simulink model "HQEV_MiL_20160830_integrate"  (Simulink 8.3)
settings: Solver=FixedStepDiscrete  StartTime=0.0  StopTime=inf  FixedStep=0.01  RelTol=1e-3
PostLoadFcn:
  | , if any(exist('dsrtsu_mdlpostloadfcn', 'file') == [2, 3, 6]), try dsrtsu_mdlpostloadfcn('Execute', bdroot); catch fprintf('Error in PostLoadFcn (dsrtsu_mdlpostloadfcn) for model "%s":\n %s\n', bdroot, lasterr); end, end,
values from neighbouring files (symbols this model uses):
  Bat_C_Ah = 36    [parameter_V1.mat]
  Bat_ocv_xIndex = [5 10 20 30 40 50 60 70 80 90 95]    [parameter_V1.mat]
  Bat_ocv_z = [329 332 340 345 347 351 358 372 377 386 391]    [parameter_V1.mat]
  Bat_R_ohm_z = [4.41 3.46 1.57 1.07 0.76 0.63 0.55 0.44 0.41 0.4 0.4 3.14 ... (66 elements, 11x6)]    [parameter_V1.mat]
  Bat_SOC_Init = 90    [parameter_V1.mat]
  Env_hum_pct_Ambient = 30    [parameter_V1.mat]
  Env_Slope_deg = 0    [parameter_V1.mat]
  Env_Temp_degC_Ambient = 25    [parameter_V1.mat]
  Env_v_kmph_HWind = 0    [parameter_V1.mat]
  Reducer_F_i = 7.23    [parameter_V1.mat]
  Reducer_R_i = 7.23    [parameter_V1.mat]
  Veh =     [parameter_V1.mat]
  Veh_A_m2_Fr = 2.246    [parameter_V1.mat]
  Veh_F_Brake =     [parameter_V1.mat]
  Veh_fac_AirDrag = 0.326    [parameter_V1.mat]
  Veh_fac_WhDragFrict_0 = 0.011    [parameter_V1.mat]
  Veh_g_mps2_C = 9.81    [parameter_V1.mat]
  Veh_GainBrake =     [parameter_V1.mat]
  Veh_h_m_COGHigh = 0.5    [parameter_V1.mat]
  Veh_J_kgm2_Wh = 1.3635    [parameter_V1.mat]
  Veh_L_m_AxlBas = 2.63    [parameter_V1.mat]
  Veh_M_kg = 1427    [parameter_V1.mat]
  Veh_mu_Brake = 0.4    [parameter_V1.mat]
  Veh_mu_Tyre =     [parameter_V1.mat]
  Veh_num_FrictPair = 8    [parameter_V1.mat]
  Veh_pct_Brk = 70    [parameter_V1.mat]
  Veh_r_dyn =     [parameter_V1.mat]
  Veh_r_m_BrkDisk = 0.136    [parameter_V1.mat]
  Veh_rho_kgpm3_Air = 1.2258    [parameter_V1.mat]
undefined symbols (not defined in the file or in its folder): DiscIntNeverNeededParam, p_bool_False_M, p_bool_True_M
libraries: BaseOperationLib_Browser x38, simulink x9, DTQC_lib x1, ERR_lib x1, MQM_lib x1, PTCL_lib x1, PUD_lib x1, TQD_lib x1, TQR_lib x1, VMM_lib x1, ACCA_lib x1, BBCA_lib x1
(part 6 of 15)

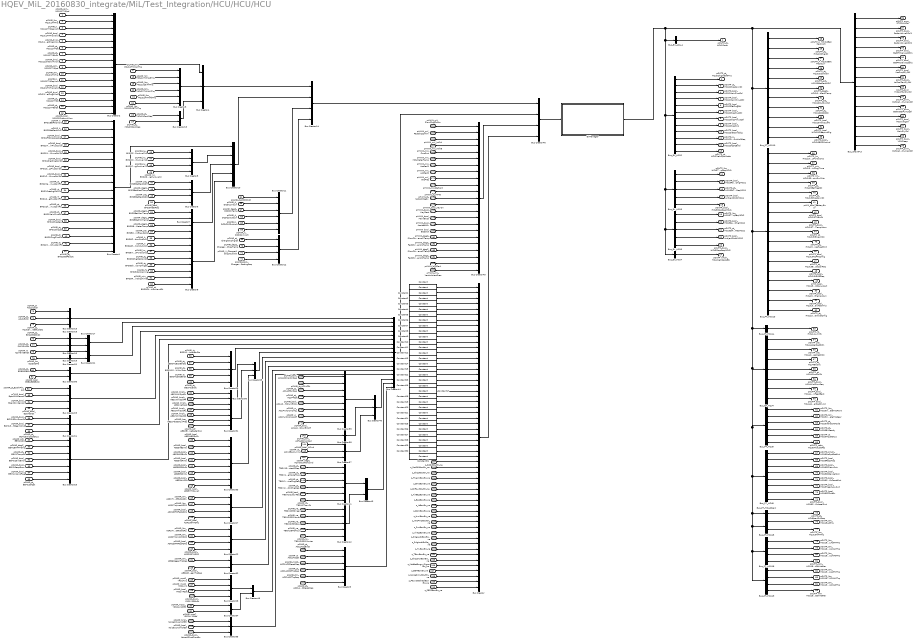
== system HQEV_MiL_20160830_integrate/MiL/Test_Integration/HCU/HCU/HCU ==
  pCANR_rpm_MCU11TMSpd : Inport
  pCANR_Nm_MCU11TMTrq : Inport  Port=2
  pCANR_V_MCU11TMCapVolt : Inport  Port=3
  pCANR_bool_MCU11TMTrqValid : Inport  Port=4
  pCANR_bool_MCU11PreChrgAllow : Inport  Port=5
  pCANR_st_MCU11TMSt : Inport  Port=6
  pCANR_st_MCU11TMErrSt : Inport  Port=7
  pCANR_bool_MCU11ShtdwnAllow : Inport  Port=8
  pCANR_rpm_MCU21TMSpd : Inport  Port=9
  pCANR_Nm_MCU21TMTrq : Inport  Port=10
  pCANR_V_MCU21TMCapVolt : Inport  Port=11
  pCANR_bool_MCU21TMTrqValid : Inport  Port=12
  pCANR_bool_MCU21PreChrgAllow : Inport  Port=13
  pCANR_st_MCU21TMSt : Inport  Port=14
  pCANR_st_MCU21TMErrSt : Inport  Port=15
  pCANR_bool_MCU21ShtdwnAllow : Inport  Port=16
  pCANR_Nm_MCU12TMMAMTrq : Inport  Port=17
  pCANR_Nm_MCU12TMMAGTrq : Inport  Port=18
  pCANR_Nm_MCU12CalTMTrq : Inport  Port=19
  pCANR_Nm_MCU22TMMAMTrq : Inport  Port=20
  pCANR_Nm_MCU22TMMAGTrq : Inport  Port=21
  pCANR_Nm_MCU22CalTMTrq : Inport  Port=22
  pCANR_st_MCU13CoolReq : Inport  Port=23
  pCANR_st_MCU23CoolReq : Inport  Port=24
  pCANR_V_BMS1BatPackVolt : Inport  Port=25
  pCANR_A_BMS1BatPackCurr : Inport  Port=26
  pCANR_bool_BMS1FltDisposeSig : Inport  Port=27
  pCANR_bool_BMS1MainPlusCoilSt : Inport  Port=28
  pCANR_bool_BMS1MainMinusCoilSt : Inport  Port=29
  pCANR_bool_BMS1PreChrgCoilSt : Inport  Port=30
  pCANR_bool_BMS1ChrgPlusCoilSt : Inport  Port=31
  pCANR_bool_BMS1ChrgMinusCoilSt : Inport  Port=32
  pCANR_st_BMS1MainMinusCoilFlt : Inport  Port=33
  pCANR_st_BMS1PrechrgCoilFlt : Inport  Port=34
  pCANR_st_BMS1ChrgPlusCoilFlt : Inport  Port=35
  pCANR_st_BMS1ChrgMinusCoilFlt : Inport  Port=36
  pCANR_st_BMS1MainPlusFlt : Inport  Port=37
  pCANR_bool_BMS1ChrgReq : Inport  Port=38
  pCANR_st_BMS1ChrgSt : Inport  Port=39
  pCANR_st_BMS1ChrgPlusFlt : Inport  Port=40
  pCANR_st_BMS1MainPlusCoilFlt : Inport  Port=41
  pCANR_st_BMS1BatPackSt : Inport  Port=42
  pCANR_kw_BMS2ChrgPwrAvail10 : Inport  Port=43
  pCANR_kw_BMS2DischrgPwrAvail10 : Inport  Port=44
  pCANR_kw_BMS2ChrgPwrAvail2 : Inport  Port=45
  pCANR_kw_BMS2DischrgPwrAvail2 : Inport  Port=46
  pCANR_pct_BMS3BatPackSOH : Inport  Port=47
  pCANR_degC_BMS3BatPackTemp : Inport  Port=48
  pCANR_pct_BMS3BatPackSOC : Inport  Port=49
  pCANR_bool_BMS3HeatReq : Inport  Port=50
  pCANR_degC_BMS5BatMaxTemp : Inport  Port=51
  pCANR_degC_BMS5BatMinTemp : Inport  Port=52
  pCANR_degC_BMS5BatInWaterTemp : Inport  Port=53
  pCANR_pct_BMS5RemainEngyRatio : Inport  Port=54
  pCANR_A_BMS6ChrgStationOutCurr : Inport  Port=55
  pCANR_V_BMS6ChrgStationOutVolt : Inport  Port=56
  pCANR_kw_BMS6InstnsPwrCnsmp : Inport  Port=57
  pCANR_st_BMS5ChrgStationSt : Inport  Port=58
  pCANR_st_BMS6ChrgStationCnfigSt : Inport  Port=59
  pCANR_st_BMS5IslaWarning : Inport  Port=60
  pCANR_min_BMS5RemainChrgTime : Inport  Port=61
  pCANR_st_BMS5ChrgStationHandSt : Inport  Port=62
  pCANR_A_DCDC1OutCurr : Inport  Port=63
  pCANR_st_DCDC1St : Inport  Port=64
  pCANR_V_DCDC1COutVolt : Inport  Port=65
  pCANR_A_DCDC1InCurr : Inport  Port=66
  pCANR_degC_DCDC1Temp : Inport  Port=67
  pCANR_V_DCDC1InVolt : Inport  Port=68
  pCANR_st_Charger1ChrgrSt : Inport  Port=69
  pCANR_degC_Charger1ChrgrTemp : Inport  Port=70
  pCANR_V_Charger1ChrgrOutVolt : Inport  Port=71
  pCANR_bool_Charger1RechrgReq : Inport  Port=72
  pCANR_st_ACU1Crash : Inport  Port=73
  pCANR_st_ACU1ErrSt : Inport  Port=74
  pCANR_st_ACU1DrvSideBuckSts : Inport  Port=75
  pCANR_st_EPS1EPSErrSt : Inport  Port=76
  pCANR_st_SAS1SASSt : Inport  Port=77
  pCANR_st_IC1HandBrkSt : Inport  Port=78
  pCANR_km_IC2DDSPS : Inport  Port=79
  pCANR_st_EPB1EPBSt : Inport  Port=80
  pCANR_bool_EPB1EPBErrSt : Inport  Port=81
  pCANR_st_EparkPrkLock : Inport  Port=82
  pCANR_bool_EparkPrkSensor : Inport  Port=83
  pCANR_bool_EparkDrvSensor : Inport  Port=84
  pCANR_bool_EparkErrSt : Inport  Port=85
  pCANR_bool_BCM13DrvDoorSt : Inport  Port=86
  pCANR_bool_BCM13HighBeamCmd : Inport  Port=87
  pCANR_st_BCM13WiperStatus : Inport  Port=88
  pCANR_pct_EEM1SOC : Inport  Port=89
  pCANR_degC_EEM1BATTTemp : Inport  Port=90
  pCANR_st_EEM1TempSt : Inport  Port=91
  pCANR_bool_EEM1CalibError : Inport  Port=92
  pCANR_bool_EEM1RespError : Inport  Port=93
  pCANR_bool_EEM1InconsFlag : Inport  Port=94
  pCANR_st_EEM1SOCSt : Inport  Port=95
  pCANR_st_EGSM1PrkLockBtnSts : Inport  Port=96
  pCANR_st_EGSM1EcoBtnSts : Inport  Port=97
  pCANR_st_EGSM1SBW1LvlPstn : Inport  Port=98
  pCANR_st_EGSM1SecBtnSt : Inport  Port=99
  pCANR_st_EGSM1ErrSt : Inport  Port=100
  pCANR_kmph_ABS1WhlSpdFL : Inport  Port=101
  pCANR_kmph_ABS1WhlSpdFR : Inport  Port=102
  pCANR_kmph_ABS1VehSpd : Inport  Port=103
  pCANR_kmph_ABS2WhlSpdRL : Inport  Port=104
  pCANR_kmph_ABS2WhlSpdRR : Inport  Port=105
  pCANR_bar_ABS2MasterCylPres : Inport  Port=106
  pCANR_pct_ABS2BrakePedalPos : Inport  Port=107
  pCANR_bool_ABS3ABSErrSt : Inport  Port=108
  pCANR_bool_ABS3ABSIntv : Inport  Port=109
  pCANR_bool_ABS3ASRErrSt : Inport  Port=110
  pCANR_bool_ABS3ASRIntv : Inport  Port=111
  pCANR_bool_ABS3ESPErrSt : Inport  Port=112
  pCANR_bool_ABS3ESPIntv : Inport  Port=113
  pCANR_bool_ABS3HHCSt : Inport  Port=114
  pCANR_bool_ABS3HHCAvail : Inport  Port=115
  pCANR_Nm_ASR1TrqRdctFastASR1 : Inport  Port=116
  pCANR_Nm_ASR1TrqIncrsMSR1 : Inport  Port=117
  pCANR_bool_ASR1StTRFastASR1 : Inport  Port=118
  pCANR_bool_ASR1StTIMSR1 : Inport  Port=119
  pCANR_Nm_ASR2TrqRdctFastASR2 : Inport  Port=120
  pCANR_Nm_ASR2TrqIncrsMSR2 : Inport  Port=121
  pCANR_bool_ASR2StTRFastASR2 : Inport  Port=122
  pCANR_bool_ASR2StTIMSR2 : Inport  Port=123
  pCANR_Nm_ABS6RegenTrqReq : Inport  Port=124
  pCANR_bool_ABS6StRegenTrqReq : Inport  Port=125
  pCANR_mps2_YRS1AX1 : Inport  Port=126
  pCANR_mps2_YRS1AY1 : Inport  Port=127
  pCANR_bool_YRS1YRSSt : Inport  Port=128
  pCANR_bool_YRS1YRSErrSt : Inport  Port=129
  pCANR_mps2_YRS2AX1Ofst : Inport  Port=130
  pCANR_mps2_YRS2AY1Ofst : Inport  Port=131
  pCANR_bool_Noise1OverVoltErr : Inport  Port=132
  pCANR_bool_Noise1UndrVoltErr : Inport  Port=133
  pCANR_bool_Noise1ShotCicutErr : Inport  Port=134
  pCANR_bool_AC1ACCmprOnReq : Inport  Port=135
  pCANR_st_AC1ACSt : Inport  Port=136
  pCANR_st_AC1ACFanReq : Inport  Port=137
  pCANR_st_AC1PTCSt : Inport  Port=138
  pCANR_bool_AC1ACShtDwnEnblL : Inport  Port=139
  pCANR_w_AC1PwrCnsmpACL : Inport  Port=140
  pCANR_w_AC1PwrCnsmpACH : Inport  Port=141
  pCANR_bool_AC1ACShtDwnEnblH : Inport  Port=142
  pCANR_rpm_ACTestCmprSpd : Inport  Port=143
  pCANR_bool_ACInd : Inport  Port=144
  pCANR_st_ACIndBLWLvlInd : Inport  Port=145
  pCANR_degC_ACIndOutTempInd : Inport  Port=146
  pCANR_st_TBOX1RemoteACReq : Inport  Port=147
  pCANR_st_TBOX1ChrgModeTbox : Inport  Port=148
  pCANR_st_TBOX1TimeChrgReq : Inport  Port=149
  pCANR_st_TBOX1InstnChrgReq : Inport  Port=150
  pCANR_bool_TBOX1QueryReq : Inport  Port=151
  pCANR_st_TBOX1TboxSt : Inport  Port=152
  pCANR_na_TBOX2GPSYear : Inport  Port=153
  pCANR_na_TBOX2GPSMonth : Inport  Port=154
  pCANR_na_TBOX2GPSDay : Inport  Port=155
  pCANR_na_TBOX2GPSHour : Inport  Port=156
  pCANR_na_TBOX2GPSMinute : Inport  Port=157
  pCANR_st_ACC1ACCErrSt : Inport  Port=158
  pCANR_st_ACC1ACCSt : Inport  Port=159
  pCANR_mps2_ACC1ACCDecelReq : Inport  Port=160
  pCANR_st_ACC1ACCStTrqReq : Inport  Port=161
  pCANR_Nm_ACC1ACCTrqReq : Inport  Port=162
  pCANR_st_ACC1ACCStACCDecelReq : Inport  Port=163
  pHWIN_mV_SlowChrgCnfrm : Inport  Port=164
  pHWIN_mV_FastChrgCnfrm : Inport  Port=165
  pHWIN_mV_IntlkA : Inport  Port=166
  pHWIN_mV_IntlkB : Inport  Port=167
  pHWIN_mV_CruzSwt : Inport  Port=168
  pHWIN_mV_MCUWaterTemp : Inport  Port=169
  pHWIN_mV_AccPed1 : Inport  Port=170
  pHWIN_mV_AccPed2 : Inport  Port=171
  pHWIN_mV_VacPres : Inport  Port=172
  pHWIN_mV_BatVolt : Inport  Port=173
  pHWIN_st_IMMO : Inport  Port=174
  pHWIN_st_NoCANMsgRx : Inport  Port=175
  pHWIN_bool_KeyOn : Inport  Port=176
  pHWIN_bool_KeyStart : Inport  Port=177
  pHWIN_bool_MainBrkSt : Inport  Port=178
  pHWIN_bool_AssistBrkSt : Inport  Port=179
  pHWIN_bool_ECOSwt : Inport  Port=180
  pHWIN_degC_SlowChrgSensr1Temp : Inport  Port=181
  pHWIN_degC_FastChrgSensr1Temp : Inport  Port=182
  pHWIN_degC_SlowChrgSensr2Temp : Inport  Port=183
  pHWIN_degC_FastChrgSensr2Temp : Inport  Port=184
  pHWIN_st_EPark : Inport  Port=185
  pHWIN_mV_VacAmbientPres : Inport  Port=186
  s_DcDcBswErr_na : Inport  Port=187
  s_MotCtlrBswErr_na : Inport  Port=188
  s_ChrgrBswErr_na : Inport  Port=189
  s_ThermBswErr_na : Inport  Port=190
  s_BmsBswErr_na : Inport  Port=191
  s_ShftLvrBswErr_na : Inport  Port=192
  s_AirBagBswErr_na : Inport  Port=193
  s_EpsBswErr_na : Inport  Port=194
  s_IcBswErr_na : Inport  Port=195
  s_BcmBswErr_na : Inport  Port=196
  s_HmiBswErr_na : Inport  Port=197
  s_VacPmpBswErr_na : Inport  Port=198
  s_PwrBswErr_na : Inport  Port=199
  s_VirtIgBswErr_na : Inport  Port=200
  s_PrkgLockBswErr_na : Inport  Port=201
  s_PrkgLockErrSts_na : Inport  Port=202
  s_HvBswErr_na : Inport  Port=203
  s_TBoxBswErr_na : Inport  Port=204
  s_ChrgSnsrBswErr_na : Inport  Port=205
  s_MotBatEmgcySignalErr_na : Inport  Port=206
  s_EEMBswErr_na : Inport  Port=207
  s_NoiseSimuBswErr_na : Inport  Port=208
  s_PasvStaCheckBswErr_na : Inport  Port=209
  s_PEPSBswErr_na : Inport  Port=210
  Bus Creator : BusCreator  Inputs=56
  Bus Creator1 : BusCreator  Inputs=18
  Bus Creator10 : BusCreator  Inputs=5
  Bus Creator{3,9,11,41} (4 alike) : BusCreator  Inputs=6
  Bus Creator{5..7,12,14,22..23,27..28,31,46} (11 alike) : BusCreator
  Bus Creator{13,17,21,32,34,36,43,48} (8 alike) : BusCreator  Inputs=2
  Bus Creator{4,15,24,29..30,35,37,40} (8 alike) : BusCreator  Inputs=3
  Bus Creator{16,18..20,38} (5 alike) : BusCreator  Inputs=1
  Bus Creator2 : BusCreator  Inputs=16
  Bus Creator25 : BusCreator  Inputs=7
  Bus Creator26 : BusCreator  Inputs=5
  Bus Creator33 : BusCreator  Inputs=8
  Bus Creator39 : BusCreator  Inputs=8
  Bus Creator42 : BusCreator  Inputs=5
  Bus Creator44 : BusCreator  Inputs=17
  Bus Creator45 : BusCreator  Inputs=23
  Bus Creator8 : BusCreator  Inputs=8
  Bus_EV_ACU_1 : BusSelector  OutputSignals=CAN_EV_BUS.pOUTP_st_ACU1Crash
  Bus_EV_HCU2 : BusSelector  OutputSignals=CAN_EV_BUS.pOUTP_st_HCU2ChrgHeatPms,CAN_EV_BUS.pOUTP_st_HCU2ChrgConnSt,CAN_EV_BUS.pOUTP_bool_HCU2MainPlusCtrl,CAN_EV_BUS.pOUTP_bool_HCU2MainMinusCtrl,CAN_EV_BUS.pOUTP_bool_HCU2PreChrgCtrl,CAN_EV_BUS.pOUTP_bool_HCU2ChrgPlusCtrl,CAN_EV_BUS.pOUTP_bool_HCU2ChrgMinusCtrl,CAN_EV_BUS.pOUTP_bool_HCU2ChrgPms,CAN_EV_BUS.pOUTP_bool_HCU2SleepIndSig,CAN_EV_BUS.pOUTP_V_HCU2DCDCOutVoltReq,CAN_EV_BUS.pOUTP_bool_HCU2DCDCEnbl,CAN_EV_BUS.pOUTP_st_HCU2VehOprtMode
  Bus_EV_HCU3 : BusSelector  OutputSignals=CAN_EV_BUS.pOUTP_Nm_HCU3TMTrqReqMCU1,CAN_EV_BUS.pOUTP_bool_HCU3RapidDisChrgMCU1,CAN_EV_BUS.pOUTP_st_HCU3StTMReqMCU1,CAN_EV_BUS.pOUTP_bool_AntijerkDisblMCU1,CAN_EV_BUS.pOUTP_bool_HCU3StopReqMCU1
  Bus_EV_HCU4 : BusSelector  OutputSignals=CAN_EV_BUS.pOUTP_kmph_HCU4VehSpdABS
  Bus_EV_HCU5 : BusSelector  OutputSignals=CAN_EV_BUS.pOUTP_Nm_HCU3TMTrqReqMCU2,CAN_EV_BUS.pOUTP_bool_HCU3RapidDisChrgMCU2,CAN_EV_BUS.pOUTP_st_HCU3StTMReqMCU2,CAN_EV_BUS.pOUTP_bool_AntijerkDisblMCU2,CAN_EV_BUS.pOUTP_bool_HCU3StopReqMCU2
  Bus_IOOutPut : BusSelector  OutputSignals=HWO_BUS.pOUTP_pwm_PTCPWMCtrl,HWO_BUS.pOUTP_bool_RadorValve1Ctrl1,HWO_BUS.pOUTP_bool_RadorValve1Ctrl2,HWO_BUS.pOUTP_bool_BatPTCValve2Ctrl1,HWO_BUS.pOUTP_bool_BatPTCValve2Ctrl2,HWO_BUS.pOUTP_bool_VacPmpRlyCtrl,HWO_BUS.pOUTP_bool_LoCoolFanRlyCtrl,HWO_BUS.pOUTP_bool_HiCoolFanRlyCtrl,HWO_BUS.pOUTP_pwm_MotWaterPump1Ctrl,HWO_BUS.pOUTP_pwm_BatWaterPumpCtrl,HWO_BUS.pOUTP_bool_MCUVirtIgOn,HWO_BUS.pOUTP_bool_MainRlyCtrl,HWO_BUS.pOUTP_bool_VCUSleep,HWO_BUS.pOUTP_pwm_MotWaterPump2Ctrl
  Bus_PT_HCU10 : BusSelector  OutputSignals=CAN_PT_BUS.pOUTP_V_HCU10BatPackVolt,CAN_PT_BUS.pOUTP_st_HCU10ChrgrSt,CAN_PT_BUS.pOUTP_A_HCU10BatPackCurr,CAN_PT_BUS.pOUTP_st_HCU10IslaWarn,CAN_PT_BUS.pOUTP_pct_HCU10BatPackSOC,CAN_PT_BUS.pOUTP_degC_HCU10BatPackTemp,CAN_PT_BUS.pOUTP_pct_HCU10OutPwrPct,CAN_PT_BUS.pOUTP_st_HCU10DCDCSt,CAN_PT_BUS.pOUTP_bool_HCU10IntlkSysFlt,CAN_PT_BUS.pOUTP_bool_HCU10SleepIndSig,CAN_PT_BUS.pOUTP_bool_HCU10ECOSwtInd
  Bus_PT_HCU13 : BusSelector  OutputSignals=CAN_PT_BUS.pOUTP_kw_HCU13InstnsPwrCnsmp,CAN_PT_BUS.pOUTP_min_HCU13RemainChrgTime,CAN_PT_BUS.pOUTP_km_HCU13RemainDrvDist,CAN_PT_BUS.pOUTP_st_HCU13BatHeatSt,CAN_PT_BUS.pOUTP_st_HCU13ChrgConnSt,CAN_PT_BUS.pOUTP_bool_HCU13BatPackErr,CAN_PT_BUS.pOUTP_bool_HCU13TMErrSt,CAN_PT_BUS.pOUTP_bool_HCU13TMTempWarn,CAN_PT_BUS.pOUTP_st_HCU13IGKeyPstn,CAN_PT_BUS.pOUTP_st_HCU13VehDeiceHeatPmt,CAN_PT_BUS.pOUTP_bool_HCU13ACPTCCnfig,CAN_PT_BUS.pOUTP_st_HCU13BatPackCoolReq,CAN_PT_BUS.pOUTP_bool_HCU13IGOffReq,CAN_PT_BUS.pOUTP_bool_HCU13BatSOCLowAlart,CAN_PT_BUS.pOUTP_bool_HCU13BatTempWarn,CAN_PT_BUS.pOUTP_bool_HCU13RemanACOnTip,CAN_PT_BUS.pOUTP_st_HCU13NoiseVoiceCnfig
  Bus_PT_HCU14 : BusSelector  OutputSignals=CAN_PT_BUS.pOUTP_st_HCU14LvlInfo
  Bus_PT_HCU15 : BusSelector  OutputSignals=CAN_PT_BUS.pOUTP_Nm_HCU15ActTrq,CAN_PT_BUS.pOUTP_Nm_HCU15MAMTrq
  Bus_PT_HCU18 : BusSelector  OutputSignals=CAN_PT_BUS.pOUTP_Nm_HCU18MCU1ActTMTrq,CAN_PT_BUS.pOUTP_Nm_HCU18MCU1MAMTrq,CAN_PT_BUS.pOUTP_Nm_HCU18MCU1MAGTrq,CAN_PT_BUS.pOUTP_rpm_HCU18MCU1ActRev
  Bus_PT_HCU19 : BusSelector  OutputSignals=CAN_PT_BUS.pOUTP_Nm_HCU19MCU2ActTMTrq,CAN_PT_BUS.pOUTP_Nm_HCU19MCU2MAMTrq,CAN_PT_BUS.pOUTP_Nm_HCU19MCU2MAGTrq,CAN_PT_BUS.pOUTP_rpm_HCU19MCU2ActRev
  Bus_PT_HCU4 : BusSelector  OutputSignals=CAN_PT_BUS.pOUTP_pct_HCU4AccelPedPstn,CAN_PT_BUS.pOUTP_pct_HCU4CalcAccelPedPstn,CAN_PT_BUS.pOUTP_st_HCU4BrkSwt,CAN_PT_BUS.pOUTP_st_HCU4CruzCtrlSt,CAN_PT_BUS.pOUTP_bool_HCU4KickDwnReq,CAN_PT_BUS.pOUTP_bool_HCU4ACOnFeedBack,CAN_PT_BUS.pOUTP_bool_HCU4AccelPedOvrid
  Bus_PT_HCU5 : BusSelector  OutputSignals=CAN_PT_BUS.pOUTP_Nm_HCU5IndicateTrqFront,CAN_PT_BUS.pOUTP_Nm_HCU5IndicateTrqRear,CAN_PT_BUS.pOUTP_st_HCU5VehOprtMode,CAN_PT_BUS.pOUTP_st_HCU5EVReady,CAN_PT_BUS.pOUTP_st_HCU5HCUStatus,CAN_PT_BUS.pOUTP_ratio_HCU5AltitudeFac
  Bus_PT_HCU8 : BusSelector  OutputSignals=CAN_PT_BUS.pOUTP_kmph_HCU8CrsSpdSetPnt,CAN_PT_BUS.pOUTP_bool_HCU8RespACC,CAN_PT_BUS.pOUTP_bool_HCU8CCMainSwt,CAN_PT_BUS.pOUTP_bool_HCU8CCCancelSwt,CAN_PT_BUS.pOUTP_bool_HCU8CCSetOrCoastSwt,CAN_PT_BUS.pOUTP_bool_HCU8HeadwaySwt,CAN_PT_BUS.pOUTP_bool_HCU8CCSwtErr,CAN_PT_BUS.pOUTP_bool_HCU8CCRsmOrAccelSwt
  Bus_PT_HCU_Epark : BusSelector  OutputSignals=CAN_PT_BUS.pOUTP_st_HCUEparkPrkReq
  Constant{,1..31} (32 alike) : BaseOperationLib_Browser/Sources&Sinks/Constant  Value=p_bool_True_M  OutMin=[]  OutMax=[]  OutDataType=fixdt(1, 16)  ConRadixGroup=Use specified scaling  OutScaling=2^0  OutDataTypeStr=Inherit: Inherit from 'Constant value'
  EVManager : Subsystem
  pOUTP_st_ACU1Crash : Outport
  pOUTP_st_HCU2ChrgHeatPms : Outport  Port=2
  pOUTP_st_HCU2ChrgConnSt : Outport  Port=3
  pOUTP_bool_HCU2MainPlusCtrl : Outport  Port=4
  pOUTP_bool_HCU2MainMinusCtrl : Outport  Port=5
  pOUTP_bool_HCU2PreChrgCtrl : Outport  Port=6
  pOUTP_bool_HCU2ChrgPlusCtrl : Outport  Port=7
  pOUTP_bool_HCU2ChrgMinusCtrl : Outport  Port=8
  pOUTP_bool_HCU2ChrgPms : Outport  Port=9
  pOUTP_bool_HCU2SleepIndSig : Outport  Port=10
  pOUTP_V_HCU2DCDCOutVoltReq : Outport  Port=11
  pOUTP_bool_HCU2DCDCEnbl : Outport  Port=12
  pOUTP_st_HCU2VehOprtMode : Outport  Port=13
  pOUTP_Nm_HCU3TMTrqReqMCU1 : Outport  Port=14
  pOUTP_bool_HCU3RapidDisChrgMCU1 : Outport  Port=15
  pOUTP_st_HCU3StTMReqMCU1 : Outport  Port=16
  pOUTP_bool_AntijerkDisblMCU1 : Outport  Port=17
  pOUTP_bool_HCU3StopReqMCU1 : Outport  Port=18
  pOUTP_Nm_HCU3TMTrqReqMCU2 : Outport  Port=19
  pOUTP_bool_HCU3RapidDisChrgMCU2 : Outport  Port=20
  pOUTP_st_HCU3StTMReqMCU2 : Outport  Port=21
  pOUTP_bool_AntijerkDisblMCU2 : Outport  Port=22
  pOUTP_bool_HCU3StopReqMCU2 : Outport  Port=23
  pOUTP_kmph_HCU4VehSpdABS : Outport  Port=24
  pOUTP_V_HCU10BatPackVolt : Outport  Port=25
  pOUTP_st_HCU10ChrgrSt : Outport  Port=26
  pOUTP_A_HCU10BatPackCurr : Outport  Port=27
  pOUTP_st_HCU10IslaWarn : Outport  Port=28
  pOUTP_pct_HCU10BatPackSOC : Outport  Port=29
  pOUTP_degC_HCU10BatPackTemp : Outport  Port=30
  pOUTP_pct_HCU10OutPwrPct : Outport  Port=31
  pOUTP_st_HCU10DCDCSt : Outport  Port=32
  pOUTP_bool_HCU10IntlkSysFlt : Outport  Port=33
  pOUTP_bool_HCU10SleepIndSig : Outport  Port=34
  pOUTP_bool_HCU10ECOSwtInd : Outport  Port=35
  pOUTP_kw_HCU13InstnsPwrCnsmp : Outport  Port=36
  pOUTP_min_HCU13RemainChrgTime : Outport  Port=37
  pOUTP_km_HCU13RemainDrvDist : Outport  Port=38
  pOUTP_st_HCU13BatHeatSt : Outport  Port=39
  pOUTP_st_HCU13ChrgConnSt : Outport  Port=40
  pHMI_bool_BatteryError : Outport  Port=41
  pOUTP_bool_HCU13TMErrSt : Outport  Port=42
  pOUTP_bool_HCU13TMTempWarn : Outport  Port=43
  pOUTP_st_HCU13IGKeyPstn : Outport  Port=44
  pOUTP_st_HCU13VehDeiceHeatPmt : Outport  Port=45
  pOUTP_bool_HCU13ACPTCCnfig : Outport  Port=46
  pOUTP_st_HCU13BatPackCoolReq : Outport  Port=47
  pOUTP_bool_HCU13IGOffReq : Outport  Port=48
  pHMI_bool_HCU13BatSOCLowAlart : Outport  Port=49
  pOUTP_bool_HCU13BatTempWarn : Outport  Port=50
  pOUTP_bool_HCU13RemanACOnTip : Outport  Port=51
  pOUTP_st_HCU13NoiseVoiceCnfig : Outport  Port=52
  pOUTP_st_HCU14LvlInfo : Outport  Port=53
  pOUTP_pct_HCU4AccelPedPstn : Outport  Port=54
  pOUTP_pct_HCU4CalcAccelPedPstn : Outport  Port=55
  pOUTP_bool_HCU4KickDwnReq : Outport  Port=56
  pOUTP_st_HCU4BrkSwt : Outport  Port=57
  pOUTP_bool_HCU4ACOnFeedBack : Outport  Port=58
  pOUTP_st_HCU4CruzCtrlSt : Outport  Port=59
  pOUTP_bool_HCU4AccelPedOvrid : Outport  Port=60
  pOUTP_Nm_HCU5IndicateTrqFront : Outport  Port=61
  pOUTP_Nm_HCU5IndicateTrqRear : Outport  Port=62
  pOUTP_st_HCU5VehOprtMode : Outport  Port=63
  pOUTP_st_HCU5EVReady : Outport  Port=64
  pOUTP_st_HCU5HCUStatus : Outport  Port=65
  pOUTP_ratio_HCU5AltitudeFac : Outport  Port=66
  pOUTP_kmph_HCU8CrsSpdSetPnt : Outport  Port=67
  pOUTP_bool_HCU8RespACC : Outport  Port=68
  pOUTP_bool_HCU8CCMainSwt : Outport  Port=69
  pOUTP_bool_HCU8CCCancelSwt : Outport  Port=70
  pOUTP_bool_HCU8CCSetOrCoastSwt : Outport  Port=71
  pOUTP_bool_HCU8HeadwaySwt : Outport  Port=72
  pOUTP_bool_HCU8CCSwtErr : Outport  Port=73
  pOUTP_bool_HCU8CCRsmOrAccelSwt : Outport  Port=74
  pOUTP_st_HCUEparkPrkReq : Outport  Port=75
  pOUTP_Nm_HCU15ActTrq : Outport  Port=76
  pOUTP_Nm_HCU15MAMTrq : Outport  Port=77
  pOUTP_Nm_HCU18MCU1ActTMTrq : Outport  Port=78
  pOUTP_Nm_HCU18MCU1MAMTrq : Outport  Port=79
  pOUTP_Nm_HCU18MCU1MAGTrq : Outport  Port=80
  pOUTP_rpm_HCU18MCU1MotCtrlActRev : Outport  Port=81
  pOUTP_Nm_HCU19MCU2ActTMTrq : Outport  Port=82
  pOUTP_Nm_HCU19MCU2MAMTrq : Outport  Port=83
  pOUTP_Nm_HCU19MCU2MAGTrq : Outport  Port=84
  pOUTP_rpm_HCU19MCU2MotCtrlActRev : Outport  Port=85
  pOUTP_pwm_PTCPWMCtrl : Outport  Port=86
  pOUTP_bool_RadorValve1Ctrl1 : Outport  Port=87
  pOUTP_bool_RadorValve1Ctrl2 : Outport  Port=88
  pOUTP_bool_BatPTCValve2Ctrl1 : Outport  Port=89
  pOUTP_bool_BatPTCValve2Ctrl2 : Outport  Port=90
  pOUTP_bool_VacPmpRlyCtrl : Outport  Port=91
  pOUTP_bool_LoCoolFanRlyCtrl : Outport  Port=92
  pOUTP_bool_HiCoolFanRlyCtrl : Outport  Port=93
  pOUTP_pwm_MotWaterPump1Ctrl : Outport  Port=94
  pOUTP_pwm_BatWaterPumpCtrl : Outport  Port=95
  pOUTP_bool_MCUVirtIgOn : Outport  Port=96
  pOUTP_bool_MainRlyCtrl : Outport  Port=97
  pOUTP_bool_VCUSleep : Outport  Port=98
  pOUTP_pwm_MotWaterPump2Ctrl : Outport  Port=99
  wires:
  Bus_PT_HCU13/14 -> pHMI_bool_HCU13BatSOCLowAlart/1  "<pOUTP_bool_HCU13BatSOCLowAlart>"
  Bus_PT_HCU13/10 -> pOUTP_st_HCU13VehDeiceHeatPmt/1  "<pOUTP_st_HCU13VehDeiceHeatPmt>"
  Bus_PT_HCU13/13 -> pOUTP_bool_HCU13IGOffReq/1  "<pOUTP_bool_HCU13IGOffReq>"
  Bus_PT_HCU13/12 -> pOUTP_st_HCU13BatPackCoolReq/1  "<pOUTP_st_HCU13BatPackCoolReq>"
  Bus_PT_HCU13/11 -> pOUTP_bool_HCU13ACPTCCnfig/1  "<pOUTP_bool_HCU13ACPTCCnfig>"
  Bus_IOOutPut/13 -> pOUTP_bool_VCUSleep/1  "<pOUTP_bool_VCUSleep>"
  Bus_IOOutPut/12 -> pOUTP_bool_MainRlyCtrl/1  "<pOUTP_bool_MainRlyCtrl>"
  Bus_IOOutPut/11 -> pOUTP_bool_MCUVirtIgOn/1  "<pOUTP_bool_MCUVirtIgOn>"
  Bus_IOOutPut/10 -> pOUTP_pwm_BatWaterPumpCtrl/1  "<pOUTP_pwm_BatWaterPumpCtrl>"
  Bus_IOOutPut/9 -> pOUTP_pwm_MotWaterPump1Ctrl/1  "<pOUTP_pwm_MotWaterPump1Ctrl>"
  Bus_IOOutPut/8 -> pOUTP_bool_HiCoolFanRlyCtrl/1  "<pOUTP_bool_HiCoolFanRlyCtrl>"
  Bus_IOOutPut/7 -> pOUTP_bool_LoCoolFanRlyCtrl/1  "<pOUTP_bool_LoCoolFanRlyCtrl>"
  Bus_IOOutPut/6 -> pOUTP_bool_VacPmpRlyCtrl/1  "<pOUTP_bool_VacPmpRlyCtrl>"
  Bus_IOOutPut/2 -> pOUTP_bool_RadorValve1Ctrl1/1  "<pOUTP_bool_RadorValve1Ctrl1>"
  Bus_IOOutPut/3 -> pOUTP_bool_RadorValve1Ctrl2/1  "<pOUTP_bool_RadorValve1Ctrl2>"
  Bus_IOOutPut/4 -> pOUTP_bool_BatPTCValve2Ctrl1/1  "<pOUTP_bool_BatPTCValve2Ctrl1>"
  Bus_IOOutPut/5 -> pOUTP_bool_BatPTCValve2Ctrl2/1  "<pOUTP_bool_BatPTCValve2Ctrl2>"
  Bus_IOOutPut/1 -> pOUTP_pwm_PTCPWMCtrl/1  "<pOUTP_pwm_PTCPWMCtrl>"
  Bus_PT_HCU_Epark/1 -> pOUTP_st_HCUEparkPrkReq/1  "<pOUTP_st_HCUEparkPrkReq>"
  Bus_PT_HCU8/1 -> pOUTP_kmph_HCU8CrsSpdSetPnt/1  "<pOUTP_kmph_HCU8CrsSpdSetPnt>"
  Bus_PT_HCU4/4 -> pOUTP_st_HCU4CruzCtrlSt/1  "<pOUTP_st_HCU4CruzCtrlSt>"
  Bus_PT_HCU4/2 -> pOUTP_pct_HCU4CalcAccelPedPstn/1  "<pOUTP_pct_HCU4CalcAccelPedPstn>"
  Bus_PT_HCU4/1 -> pOUTP_pct_HCU4AccelPedPstn/1  "<pOUTP_pct_HCU4AccelPedPstn>"
  Bus_PT_HCU5/3 -> pOUTP_st_HCU5VehOprtMode/1  "<pOUTP_st_HCU5VehOprtMode>"
  Bus_PT_HCU5/4 -> pOUTP_st_HCU5EVReady/1  "<pOUTP_st_HCU5EVReady>"
  Bus_PT_HCU5/5 -> pOUTP_st_HCU5HCUStatus/1  "<pOUTP_st_HCU5HCUStatus>"
  Bus_PT_HCU14/1 -> pOUTP_st_HCU14LvlInfo/1  "<pOUTP_st_HCU14LvlInfo>"
  Bus_PT_HCU13/8 -> pOUTP_bool_HCU13TMTempWarn/1  "<pOUTP_bool_HCU13TMTempWarn>"
  Bus_PT_HCU13/9 -> pOUTP_st_HCU13IGKeyPstn/1  "<pOUTP_st_HCU13IGKeyPstn>"
  Bus_PT_HCU13/6 -> pHMI_bool_BatteryError/1  "<pOUTP_bool_HCU13BatPackErr>"
  Bus_PT_HCU13/3 -> pOUTP_km_HCU13RemainDrvDist/1  "<pOUTP_km_HCU13RemainDrvDist>"
  Bus_PT_HCU13/1 -> pOUTP_kw_HCU13InstnsPwrCnsmp/1  "<pOUTP_kw_HCU13InstnsPwrCnsmp>"
  Bus_PT_HCU13/2 -> pOUTP_min_HCU13RemainChrgTime/1  "<pOUTP_min_HCU13RemainChrgTime>"
  Bus_PT_HCU13/4 -> pOUTP_st_HCU13BatHeatSt/1  "<pOUTP_st_HCU13BatHeatSt>"
  Bus_PT_HCU13/5 -> pOUTP_st_HCU13ChrgConnSt/1  "<pOUTP_st_HCU13ChrgConnSt>"
  Bus_PT_HCU10/11 -> pOUTP_bool_HCU10ECOSwtInd/1  "<pOUTP_bool_HCU10ECOSwtInd>"
  Bus_PT_HCU10/10 -> pOUTP_bool_HCU10SleepIndSig/1  "<pOUTP_bool_HCU10SleepIndSig>"
  Bus_PT_HCU10/1 -> pOUTP_V_HCU10BatPackVolt/1  "<pOUTP_V_HCU10BatPackVolt>"
  Bus_PT_HCU10/2 -> pOUTP_st_HCU10ChrgrSt/1  "<pOUTP_st_HCU10ChrgrSt>"
  Bus_PT_HCU10/3 -> pOUTP_A_HCU10BatPackCurr/1  "<pOUTP_A_HCU10BatPackCurr>"
  Bus_PT_HCU10/4 -> pOUTP_st_HCU10IslaWarn/1  "<pOUTP_st_HCU10IslaWarn>"
  Bus_PT_HCU10/5 -> pOUTP_pct_HCU10BatPackSOC/1  "<pOUTP_pct_HCU10BatPackSOC>"
  Bus_PT_HCU10/6 -> pOUTP_degC_HCU10BatPackTemp/1  "<pOUTP_degC_HCU10BatPackTemp>"
  Bus_PT_HCU10/7 -> pOUTP_pct_HCU10OutPwrPct/1  "<pOUTP_pct_HCU10OutPwrPct>"
  Bus_PT_HCU10/8 -> pOUTP_st_HCU10DCDCSt/1  "<pOUTP_st_HCU10DCDCSt>"
  Bus_PT_HCU10/9 -> pOUTP_bool_HCU10IntlkSysFlt/1  "<pOUTP_bool_HCU10IntlkSysFlt>"
  Bus_EV_HCU4/1 -> pOUTP_kmph_HCU4VehSpdABS/1  "<pOUTP_kmph_HCU4VehSpdABS>"
  Bus_EV_HCU3/4 -> pOUTP_bool_AntijerkDisblMCU1/1  "<pOUTP_bool_AntijerkDisblMCU1>"
  Bus_EV_HCU3/3 -> pOUTP_st_HCU3StTMReqMCU1/1  "<pOUTP_st_HCU3StTMReqMCU1>"
  Bus_EV_HCU3/2 -> pOUTP_bool_HCU3RapidDisChrgMCU1/1  "<pOUTP_bool_HCU3RapidDisChrgMCU1>"
  Bus_EV_HCU3/1 -> pOUTP_Nm_HCU3TMTrqReqMCU1/1  "<pOUTP_Nm_HCU3TMTrqReqMCU1>"
  Bus_EV_HCU2/12 -> pOUTP_st_HCU2VehOprtMode/1  "<pOUTP_st_HCU2VehOprtMode>"
  Bus_EV_HCU2/11 -> pOUTP_bool_HCU2DCDCEnbl/1  "<pOUTP_bool_HCU2DCDCEnbl>"
  Bus_EV_HCU2/10 -> pOUTP_V_HCU2DCDCOutVoltReq/1  "<pOUTP_V_HCU2DCDCOutVoltReq>"
  Bus_EV_HCU2/9 -> pOUTP_bool_HCU2SleepIndSig/1  "<pOUTP_bool_HCU2SleepIndSig>"
  Bus_EV_HCU2/6 -> pOUTP_bool_HCU2ChrgPlusCtrl/1  "<pOUTP_bool_HCU2ChrgPlusCtrl>"
  Bus_EV_HCU2/7 -> pOUTP_bool_HCU2ChrgMinusCtrl/1  "<pOUTP_bool_HCU2ChrgMinusCtrl>"
  Bus_EV_HCU2/3 -> pOUTP_bool_HCU2MainPlusCtrl/1  "<pOUTP_bool_HCU2MainPlusCtrl>"
  Bus_EV_HCU2/8 -> pOUTP_bool_HCU2ChrgPms/1  "<pOUTP_bool_HCU2ChrgPms>"
  Bus_EV_HCU2/5 -> pOUTP_bool_HCU2PreChrgCtrl/1  "<pOUTP_bool_HCU2PreChrgCtrl>"
  Bus_EV_HCU2/4 -> pOUTP_bool_HCU2MainMinusCtrl/1  "<pOUTP_bool_HCU2MainMinusCtrl>"
  Bus_EV_HCU2/2 -> pOUTP_st_HCU2ChrgConnSt/1  "<pOUTP_st_HCU2ChrgConnSt>"
  Bus_EV_ACU_1/1 -> pOUTP_st_ACU1Crash/1  "<pOUTP_st_ACU1Crash>"
  Bus_EV_HCU2/1 -> pOUTP_st_HCU2ChrgHeatPms/1  "<pOUTP_st_HCU2ChrgHeatPms>"
  EVManager/1(RTEOut) -> Bus_PT_HCU10/1, Bus_PT_HCU13/1, Bus_PT_HCU14/1, Bus_PT_HCU4/1, Bus_PT_HCU5/1, Bus_PT_HCU8/1, Bus_PT_HCU_Epark/1, Bus_PT_HCU15/1, Bus_PT_HCU18/1, Bus_PT_HCU19/1, Bus_IOOutPut/1, Bus_EV_ACU_1/1, Bus_EV_HCU2/1, Bus_EV_HCU5/1, Bus_EV_HCU4/1, Bus_EV_HCU3/1
  pCANR_V_BMS1BatPackVolt/1 -> Bus Creator1/1  "pCANR_V_BMS1BatPackVolt"
  pCANR_A_BMS1BatPackCurr/1 -> Bus Creator1/2  "pCANR_A_BMS1BatPackCurr"
  pCANR_bool_BMS1MainPlusCoilSt/1 -> Bus Creator1/4  "pCANR_bool_BMS1MainPlusCoilSt"
  pCANR_bool_BMS1MainMinusCoilSt/1 -> Bus Creator1/5  "pCANR_bool_BMS1MainMinusCoilSt"
  pCANR_bool_BMS1PreChrgCoilSt/1 -> Bus Creator1/6  "pCANR_bool_BMS1PreChrgCoilSt"
  pCANR_bool_BMS1ChrgReq/1 -> Bus Creator1/14  "pCANR_bool_BMS1ChrgReq"
  pCANR_st_BMS1ChrgSt/1 -> Bus Creator1/15  "pCANR_st_BMS1ChrgSt"
  pCANR_st_BMS1BatPackSt/1 -> Bus Creator1/18  "pCANR_st_BMS1BatPackSt"
  pCANR_kw_BMS2ChrgPwrAvail10/1 -> Bus Creator5/1  "pCANR_kw_BMS2ChrgPwrAvail10"
  pCANR_kw_BMS2DischrgPwrAvail10/1 -> Bus Creator5/2  "pCANR_kw_BMS2DischrgPwrAvail10"
  pCANR_kw_BMS2DischrgPwrAvail2/1 -> Bus Creator5/4  "pCANR_kw_BMS2DischrgPwrAvail2"
  pCANR_pct_BMS3BatPackSOH/1 -> Bus Creator6/1  "pCANR_pct_BMS3BatPackSOH"
  pCANR_degC_BMS3BatPackTemp/1 -> Bus Creator6/2  "pCANR_degC_BMS3BatPackTemp"
  pCANR_pct_BMS3BatPackSOC/1 -> Bus Creator6/3  "pCANR_pct_BMS3BatPackSOC"
  pCANR_degC_BMS5BatMaxTemp/1 -> Bus Creator7/1  "pCANR_degC_BMS5BatMaxTemp"
  pCANR_degC_BMS5BatMinTemp/1 -> Bus Creator7/2  "pCANR_degC_BMS5BatMinTemp"
  pCANR_degC_BMS5BatInWaterTemp/1 -> Bus Creator7/3  "pCANR_degC_BMS5BatInWaterTemp"
  pCANR_st_BMS5IslaWarning/1 -> Bus Creator8/6  "pCANR_st_BMS5IslaWarning"
  pCANR_bool_BMS1FltDisposeSig/1 -> Bus Creator1/3  "pCANR_bool_BMS1FltDisposeSig"
  pCANR_bool_BMS1ChrgPlusCoilSt/1 -> Bus Creator1/7  "pCANR_bool_BMS1ChrgPlusCoilSt"
  pCANR_bool_BMS1ChrgMinusCoilSt/1 -> Bus Creator1/8  "pCANR_bool_BMS1ChrgMinusCoilSt"
  pCANR_st_BMS1MainMinusCoilFlt/1 -> Bus Creator1/9  "pCANR_st_BMS1MainMinusCoilFlt"
  pCANR_st_BMS1PrechrgCoilFlt/1 -> Bus Creator1/10  "pCANR_st_BMS1PrechrgCoilFlt"
  pCANR_st_BMS1ChrgPlusCoilFlt/1 -> Bus Creator1/11  "pCANR_st_BMS1ChrgPlusCoilFlt"
  pCANR_st_BMS1ChrgMinusCoilFlt/1 -> Bus Creator1/12  "pCANR_st_BMS1ChrgMinusCoilFlt"
  pCANR_st_BMS1MainPlusFlt/1 -> Bus Creator1/13  "pCANR_st_BMS1MainPlusFlt"
  pCANR_st_BMS1ChrgPlusFlt/1 -> Bus Creator1/16  "pCANR_st_BMS1ChrgPlusFlt"
  pCANR_st_BMS1MainPlusCoilFlt/1 -> Bus Creator1/17  "pCANR_st_BMS1MainPlusCoilFlt"
  pCANR_A_BMS6ChrgStationOutCurr/1 -> Bus Creator8/1  "pCANR_A_BMS6ChrgStationOutCurr"
  pCANR_V_BMS6ChrgStationOutVolt/1 -> Bus Creator8/2  "pCANR_V_BMS6ChrgStationOutVolt"
  pCANR_kw_BMS6InstnsPwrCnsmp/1 -> Bus Creator8/3  "pCANR_kw_BMS6InstnsPwrCnsmp"
  pCANR_st_BMS5ChrgStationSt/1 -> Bus Creator8/4  "pCANR_st_BMS5ChrgStationSt"
  pCANR_st_BMS6ChrgStationCnfigSt/1 -> Bus Creator8/5  "pCANR_st_BMS6ChrgStationCnfigSt"
  pCANR_min_BMS5RemainChrgTime/1 -> Bus Creator8/7  "pCANR_min_BMS5RemainChrgTime"
  pCANR_kw_BMS2ChrgPwrAvail2/1 -> Bus Creator5/3  "pCANR_kw_BMS2ChrgPwrAvail2"
  pCANR_bool_BMS3HeatReq/1 -> Bus Creator6/4  "pCANR_bool_BMS3HeatReq"
  pCANR_pct_BMS5RemainEngyRatio/1 -> Bus Creator7/4  "pCANR_pct_BMS5RemainEngyRatio"
  pCANR_st_BMS5ChrgStationHandSt/1 -> Bus Creator8/8  "pCANR_st_BMS5ChrgStationHandSt"
  Bus Creator1/1 -> Bus Creator10/1  "pCANR_BMS1"
  Bus Creator5/1 -> Bus Creator10/2  "pCANR_BMS2"
  Bus Creator6/1 -> Bus Creator10/3  "pCANR_BMS3"
  Bus Creator7/1 -> Bus Creator10/4  "pCANR_BMS4"
  Bus Creator8/1 -> Bus Creator10/5  "pCANR_BMS5"
  pCANR_st_DCDC1St/1 -> Bus Creator11/1  "pCANR_st_DCDC1St"
  pCANR_A_DCDC1InCurr/1 -> Bus Creator11/2  "pCANR_A_DCDC1InCurr"
  pCANR_degC_DCDC1Temp/1 -> Bus Creator11/3  "pCANR_degC_DCDC1Temp"
  pCANR_A_DCDC1OutCurr/1 -> Bus Creator11/4  "pCANR_A_DCDC1OutCurr"
  pCANR_V_DCDC1COutVolt/1 -> Bus Creator11/5  "pCANR_V_DCDC1COutVolt"
  Bus Creator11/1 -> Bus Creator14/3  "pCANR_DCDC1"
  pCANR_bool_Charger1RechrgReq/1 -> Bus Creator12/4  "pCANR_bool_Charger1RechrgReq"
  pCANR_V_Charger1ChrgrOutVolt/1 -> Bus Creator12/3  "pCANR_V_Charger1ChrgrOutVolt"
  pCANR_degC_Charger1ChrgrTemp/1 -> Bus Creator12/2  "pCANR_degC_Charger1ChrgrTemp"
  pCANR_st_Charger1ChrgrSt/1 -> Bus Creator12/1  "pCANR_st_Charger1ChrgrSt"
  Bus Creator12/1 -> Bus Creator14/4  "pCANR_Charger1"
  pCANR_V_DCDC1InVolt/1 -> Bus Creator11/6  "pCANR_V_DCDC1InVolt"
  Bus Creator4/1 -> Bus Creator14/1  "pCANR_MCU"
  Bus Creator10/1 -> Bus Creator14/2  "pCANR_BMS"
  pCANR_st_ACU1Crash/1 -> Bus Creator15/1  "pCANR_st_ACU1Crash"
  pCANR_st_ACU1ErrSt/1 -> Bus Creator15/2  "pCANR_st_ACU1ErrSt"
  Bus Creator15/1 -> Bus Creator44/1  "pCANR_Airbag1"
  pCANR_st_SAS1SASSt/1 -> Bus Creator16/1  "pCANR_st_SAS1SASSt"
  pCANR_st_EPS1EPSErrSt/1 -> Bus Creator18/1  "pCANR_st_EPS1EPSErrSt"
  Bus Creator18/1 -> Bus Creator17/1  "pCANR_EPS1"
  Bus Creator16/1 -> Bus Creator17/2  "pCANR_SAS1"
  Bus Creator17/1 -> Bus Creator44/2  "pCANR_ESP"
  pCANR_km_IC2DDSPS/1 -> Bus Creator20/1  "pCANR_km_IC2DDSPS"
  pCANR_st_IC1HandBrkSt/1 -> Bus Creator19/1  "pCANR_st_IC1HandBrkSt"
  Bus Creator19/1 -> Bus Creator21/1  "pCANR_IC1"
  Bus Creator20/1 -> Bus Creator21/2  "pCANR_IC2"
  pCANR_bool_EparkPrkSensor/1 -> Bus Creator23/2  "pCANR_bool_EparkPrkSensor"
  pCANR_bool_EparkDrvSensor/1 -> Bus Creator23/3  "pCANR_bool_EparkDrvSensor"
  pCANR_st_EparkPrkLock/1 -> Bus Creator23/1  "pCANR_st_EparkPrkLock"
  Bus Creator23/1 -> Bus Creator44/5  "pCAN_ePark_STATE"
  pCANR_pct_EEM1SOC/1 -> Bus Creator25/1  "pCANR_pct_EEM1SOC"
  pCANR_degC_EEM1BATTTemp/1 -> Bus Creator25/2  "pCANR_degC_EEM1BATTTemp"
  pCANR_st_EEM1TempSt/1 -> Bus Creator25/3  "pCANR_st_EEM1TempSt"
  pCANR_bool_EEM1CalibError/1 -> Bus Creator25/4  "pCANR_bool_EEM1CalibError"
  pCANR_bool_EEM1RespError/1 -> Bus Creator25/5  "pCANR_bool_EEM1RespError"
  pCANR_bool_EEM1InconsFlag/1 -> Bus Creator25/6  "pCANR_bool_EEM1InconsFlag"
  pCANR_st_EEM1SOCSt/1 -> Bus Creator25/7  "pCANR_st_EEM1SOCSt"
  Bus Creator25/1 -> Bus Creator44/7  "pCANR_EEM1"
  pCANR_st_EGSM1PrkLockBtnSts/1 -> Bus Creator26/1  "pCANR_st_EGSM1PrkLockBtnSts"
  pCANR_st_EGSM1EcoBtnSts/1 -> Bus Creator26/2  "pCANR_st_EGSM1EcoBtnSts"
  pCANR_st_EGSM1SBW1LvlPstn/1 -> Bus Creator26/3  "pCANR_st_EGSM1SBW1LvlPstn"
  Bus Creator26/1 -> Bus Creator44/8  "pCANR_EGSM1"
  pCANR_bool_Noise1ShotCicutErr/1 -> Bus Creator35/3  "pCANR_bool_Noise1ShotCicutErr"
  pCANR_bool_Noise1UndrVoltErr/1 -> Bus Creator35/2  "pCANR_bool_Noise1UndrVoltErr"
  pCANR_bool_Noise1OverVoltErr/1 -> Bus Creator35/1  "pCANR_bool_Noise1OverVoltErr"
  pCANR_bool_AC1ACShtDwnEnblH/1 -> Bus Creator39/8  "pCANR_bool_AC1ACShtDwnEnblH"
  pCANR_w_AC1PwrCnsmpACH/1 -> Bus Creator39/7  "pCANR_w_AC1PwrCnsmpACH"
  pCANR_w_AC1PwrCnsmpACL/1 -> Bus Creator39/6  "pCANR_w_AC1PwrCnsmpACL"
  pCANR_bool_AC1ACShtDwnEnblL/1 -> Bus Creator39/5  "pCANR_bool_AC1ACShtDwnEnblL"
  pCANR_bool_AC1ACCmprOnReq/1 -> Bus Creator39/1  "pCANR_bool_AC1ACCmprOnReq"
  pCANR_rpm_ACTestCmprSpd/1 -> Bus Creator38/1  "pCANR_rpm_ACTestCmprSpd"
  Bus Creator37/1 -> Bus Creator40/3  "pCANR_AC1Indication"
  Bus Creator38/1 -> Bus Creator40/2  "pCANR_ACTest"
  Bus Creator39/1 -> Bus Creator40/1  "pCANR_AC1"
  pCANR_degC_ACIndOutTempInd/1 -> Bus Creator37/3  "pCANR_degC_ACIndOutTempInd"
  pCANR_st_ACIndBLWLvlInd/1 -> Bus Creator37/2  "pCANR_st_ACIndBLWLvlInd"
  pCANR_bool_ACInd/1 -> Bus Creator37/1  "pCANR_bool_ACInd"
  pCANR_st_AC1ACFanReq/1 -> Bus Creator39/3  "pCANR_st_AC1ACFanReq"
  pCANR_st_AC1ACSt/1 -> Bus Creator39/2  "pCANR_st_AC1ACSt"
  pCANR_st_AC1PTCSt/1 -> Bus Creator39/4  "pCANR_st_AC1PTCSt"
  pCANR_st_TBOX1TboxSt/1 -> Bus Creator41/6  "pCANR_st_TBOX1TboxSt"
  pCANR_bool_TBOX1QueryReq/1 -> Bus Creator41/5  "pCANR_bool_TBOX1QueryReq"
  pCANR_st_TBOX1InstnChrgReq/1 -> Bus Creator41/4  "pCANR_st_TBOX1InstnChrgReq"
  pCANR_st_TBOX1TimeChrgReq/1 -> Bus Creator41/3  "pCANR_st_TBOX1TimeChrgReq"
  pCANR_st_TBOX1ChrgModeTbox/1 -> Bus Creator41/2  "pCANR_st_TBOX1ChrgModeTbox"
  pCANR_st_TBOX1RemoteACReq/1 -> Bus Creator41/1  "pCANR_st_TBOX1RemoteACReq"
  Bus Creator41/1 -> Bus Creator43/1  "pCANR_TBOX1"
  pCANR_na_TBOX2GPSMinute/1 -> Bus Creator42/5  "pCANR_na_TBOX2GPSMinute"
  pCANR_na_TBOX2GPSHour/1 -> Bus Creator42/4  "pCANR_na_TBOX2GPSHour"
  pCANR_na_TBOX2GPSDay/1 -> Bus Creator42/3  "pCANR_na_TBOX2GPSDay"
  pCANR_na_TBOX2GPSMonth/1 -> Bus Creator42/2  "pCANR_na_TBOX2GPSMonth"
  pCANR_na_TBOX2GPSYear/1 -> Bus Creator42/1  "pCANR_na_TBOX2GPSYear"
  Bus Creator42/1 -> Bus Creator43/2  "pCANR_TBOX2"
  Bus Creator21/1 -> Bus Creator44/3  "pCANR_IC"
  pHWIN_bool_AssistBrkSt/1 -> Bus Creator45/16  "pHWIN_bool_AssistBrkSt"
  pHWIN_bool_MainBrkSt/1 -> Bus Creator45/15  "pHWIN_bool_MainBrkSt"
  pHWIN_bool_KeyStart/1 -> Bus Creator45/14  "pHWIN_bool_KeyStart"
  pHWIN_bool_KeyOn/1 -> Bus Creator45/13  "pHWIN_bool_KeyOn"
  pHWIN_st_IMMO/1 -> Bus Creator45/11  "pHWIN_st_IMMO"
  pHWIN_mV_BatVolt/1 -> Bus Creator45/10  "pHWIN_mV_BatVolt"
  pHWIN_mV_VacPres/1 -> Bus Creator45/9  "pHWIN_mV_VacPres"
  pHWIN_mV_AccPed2/1 -> Bus Creator45/8  "pHWIN_mV_AccPed2"
  pHWIN_mV_AccPed1/1 -> Bus Creator45/7  "pHWIN_mV_AccPed1"
  pHWIN_mV_MCUWaterTemp/1 -> Bus Creator45/6  "pHWIN_mV_MCUWaterTemp"
  pHWIN_mV_CruzSwt/1 -> Bus Creator45/5  "pHWIN_mV_CruzSwt"
  pHWIN_mV_IntlkB/1 -> Bus Creator45/4  "pHWIN_mV_IntlkB"
  pHWIN_mV_IntlkA/1 -> Bus Creator45/3  "pHWIN_mV_IntlkA"
  pHWIN_mV_SlowChrgCnfrm/1 -> Bus Creator45/1  "pHWIN_mV_SlowChrgCnfrm"
  pHWIN_bool_ECOSwt/1 -> Bus Creator45/17  "pHWIN_bool_ECOSwt"
  pHWIN_mV_FastChrgCnfrm/1 -> Bus Creator45/2  "pHWIN_mV_FastChrgCnfrm"
  pHWIN_st_NoCANMsgRx/1 -> Bus Creator45/12  "pHWIN_st_NoCANMsgRx"
  Bus Creator14/1 -> Bus Creator46/1  "pCANR_EV"
  Bus Creator44/1 -> Bus Creator46/2  "pCANR_PT"
  Bus Creator45/1 -> Bus Creator46/3  "IO"
  Bus Creator46/1 -> EVManager/1(RTEIn)  "RTEIn"
  Constant20/1 -> Bus Creator/23  "s_MotCpUVld_na"
  Constant19/1 -> Bus Creator/22  "s_MotCtlrCurrDrvTqLimBoostVld_na"
  Constant18/1 -> Bus Creator/21  "s_MotCtlrCurrRcpTqLimBoostVld_na"
  Constant17/1 -> Bus Creator/20  "s_MotInvActTVld_na"
  Constant16/1 -> Bus Creator/19  "s_MotCtlrActTVld_na"
  Constant23/1 -> Bus Creator/18  "s_AirCdnPwrCnsVld_na"
  Constant22/1 -> Bus Creator/17  "s_EgyCpBatVld_na"
  Constant15/1 -> Bus Creator/16  "pHWIN_bool_BatOutTVld"
  Constant14/1 -> Bus Creator/15  "pHWIN_bool_BatInpTVld"
  Constant13/1 -> Bus Creator/14  "pHWIN_bool_BatAvgTVld"
  Constant12/1 -> Bus Creator/13  "pHWIN_bool_BatMinTVld"
  Constant11/1 -> Bus Creator/12  "pHWIN_bool_BatMaxTVld"
  Constant10/1 -> Bus Creator/11  "pHWIN_bool_BatSOHVld"
  Constant9/1 -> Bus Creator/10  "pHWIN_bool_BatStOfChVld"
  Constant8/1 -> Bus Creator/9  "pHWIN_bool_BatActIVld"
  Constant7/1 -> Bus Creator/8  "pHWIN_bool_BatActUVld"
  Constant6/1 -> Bus Creator/7  "pHWIN_bool_MaxDchaPwrBoostVld"
  Constant5/1 -> Bus Creator/6  "pHWIN_bool_MaxChPwrBoostVld"
  Constant4/1 -> Bus Creator/5  "pHWIN_bool_BatMaxDchaPwrVld"
  Constant3/1 -> Bus Creator/4  "pHWIN_bool_BatMaxChPwrVld"
  Constant2/1 -> Bus Creator/3  "s_VehLgtSpdVld_na"
  Constant1/1 -> Bus Creator/2  "s_EspBswErr_na"
  Constant/1 -> Bus Creator/1  "s_ChrgrTVld_na"
  s_PwrBswErr_na/1 -> Bus Creator/45  "s_PwrBswErr_na"
  s_VacPmpBswErr_na/1 -> Bus Creator/44  "s_VacPmpBswErr_na"
  s_HmiBswErr_na/1 -> Bus Creator/43  "s_HmiBswErr_na"
  s_BcmBswErr_na/1 -> Bus Creator/42  "s_BcmBswErr_na"
  s_IcBswErr_na/1 -> Bus Creator/41  "s_IcBswErr_na"
  s_EpsBswErr_na/1 -> Bus Creator/40  "s_EpsBswErr_na"
  s_AirBagBswErr_na/1 -> Bus Creator/39  "s_AirBagBswErr_na"
  s_ShftLvrBswErr_na/1 -> Bus Creator/38  "s_ShftLvrBswErr_na"
  s_BmsBswErr_na/1 -> Bus Creator/37  "s_BmsBswErr_na"
  s_ThermBswErr_na/1 -> Bus Creator/36  "s_ThermBswErr_na"
  s_ChrgrBswErr_na/1 -> Bus Creator/35  "s_ChrgrBswErr_na"
  s_MotCtlrBswErr_na/1 -> Bus Creator/34  "s_MotCtlrBswErr_na"
  Constant26/1 -> Bus Creator/27  "s_CurAmbTVld_na"
  s_DcDcBswErr_na/1 -> Bus Creator/33  "s_DcDcBswErr_na"
  Constant25/1 -> Bus Creator/26  "s_DcDcActTVld_na"
  Constant24/1 -> Bus Creator/25  "s_DcDcActInpIVld_na"
  Constant21/1 -> Bus Creator/24  "s_ActChrgrIVld_na"
  s_HvBswErr_na/1 -> Bus Creator/49  "s_HvBswErr_na"
  s_PrkgLockErrSts_na/1 -> Bus Creator/48  "s_PrkgLockErrSts_na"
  s_PrkgLockBswErr_na/1 -> Bus Creator/47  "s_PrkgLockBswErr_na"
  s_VirtIgBswErr_na/1 -> Bus Creator/46  "s_VirtIgBswErr_na"
  Bus Creator/1 -> Bus Creator46/4  "ErrorSignal"
  pCANR_kmph_ABS1WhlSpdFR/1 -> Bus Creator30/2  "pCANR_kmph_ABS1WhlSpdFR"
  pCANR_kmph_ABS2WhlSpdRL/1 -> Bus Creator31/1  "pCANR_kmph_ABS2WhlSpdRL"
  pCANR_kmph_ABS2WhlSpdRR/1 -> Bus Creator31/2  "pCANR_kmph_ABS2WhlSpdRR"
  pCANR_mps2_YRS1AX1/1 -> Bus Creator28/1  "pCANR_mps2_YRS1AX1"
  pCANR_mps2_YRS1AY1/1 -> Bus Creator28/2  "pCANR_mps2_YRS1AY1"
  pCANR_bool_YRS1YRSSt/1 -> Bus Creator28/3  "pCANR_bool_YRS1YRSSt"
  pCANR_kmph_ABS1VehSpd/1 -> Bus Creator30/3  "pCANR_kmph_ABS1VehSpd"
  pCANR_bar_ABS2MasterCylPres/1 -> Bus Creator31/3  "pCANR_bar_ABS2MasterCylPres"
  pCANR_bool_YRS1YRSErrSt/1 -> Bus Creator28/4  "pCANR_bool_YRS1YRSErrSt"
  pCANR_kmph_ABS1WhlSpdFL/1 -> Bus Creator30/1  "pCANR_kmph_ABS1WhlSpdFL"
  pCANR_bool_ABS3ABSErrSt/1 -> Bus Creator33/1  "pCANR_bool_ABS3ABSErrSt"
  pCANR_bool_ABS3ABSIntv/1 -> Bus Creator33/2  "pCANR_bool_ABS3ABSIntv"
  pCANR_bool_ABS3ASRErrSt/1 -> Bus Creator33/3  "pCANR_bool_ABS3ASRErrSt"
  pCANR_bool_ABS3ASRIntv/1 -> Bus Creator33/4  "pCANR_bool_ABS3ASRIntv"
  pCANR_bool_ABS3ESPErrSt/1 -> Bus Creator33/5  "pCANR_bool_ABS3ESPErrSt"
  pCANR_bool_ABS3ESPIntv/1 -> Bus Creator33/6  "pCANR_bool_ABS3ESPIntv"
  pCANR_bool_ABS3HHCSt/1 -> Bus Creator33/7  "pCANR_bool_ABS3HHCSt"
  Bus Creator30/1 -> Bus Creator29/1  "pCANR_ABS1"
  Bus Creator31/1 -> Bus Creator29/2  "pCANR_ABS2"
  Bus Creator33/1 -> Bus Creator29/3  "pCANR_ABS3"
  Bus Creator28/1 -> Bus Creator48/1  "pCANR_YRS1"
  Bus Creator27/1 -> Bus Creator44/10  "pCANR_ASR1"
  Bus Creator29/1 -> Bus Creator44/9  "pCANR_ABS"
  Bus_EV_HCU5/1 -> pOUTP_Nm_HCU3TMTrqReqMCU2/1  "<pOUTP_Nm_HCU3TMTrqReqMCU2>"
  Bus_EV_HCU5/2 -> pOUTP_bool_HCU3RapidDisChrgMCU2/1  "<pOUTP_bool_HCU3RapidDisChrgMCU2>"
  Bus_EV_HCU5/3 -> pOUTP_st_HCU3StTMReqMCU2/1  "<pOUTP_st_HCU3StTMReqMCU2>"
  Bus_EV_HCU5/4 -> pOUTP_bool_AntijerkDisblMCU2/1  "<pOUTP_bool_AntijerkDisblMCU2>"
  Bus_EV_HCU3/5 -> pOUTP_bool_HCU3StopReqMCU1/1  "<pOUTP_bool_HCU3StopReqMCU1>"
  Bus_EV_HCU5/5 -> pOUTP_bool_HCU3StopReqMCU2/1  "<pOUTP_bool_HCU3StopReqMCU2>"
  Bus_IOOutPut/14 -> pOUTP_pwm_MotWaterPump2Ctrl/1  "<pOUTP_pwm_MotWaterPump2Ctrl>"
  Bus_PT_HCU8/2 -> pOUTP_bool_HCU8RespACC/1  "<pOUTP_bool_HCU8RespACC>"
  Bus_PT_HCU8/3 -> pOUTP_bool_HCU8CCMainSwt/1  "<pOUTP_bool_HCU8CCMainSwt>"
  Bus_PT_HCU8/4 -> pOUTP_bool_HCU8CCCancelSwt/1  "<pOUTP_bool_HCU8CCCancelSwt>"
  Bus_PT_HCU8/5 -> pOUTP_bool_HCU8CCSetOrCoastSwt/1  "<pOUTP_bool_HCU8CCSetOrCoastSwt>"
  Bus_PT_HCU8/6 -> pOUTP_bool_HCU8HeadwaySwt/1  "<pOUTP_bool_HCU8HeadwaySwt>"
  Bus_PT_HCU8/7 -> pOUTP_bool_HCU8CCSwtErr/1  "<pOUTP_bool_HCU8CCSwtErr>"
  Bus_PT_HCU8/8 -> pOUTP_bool_HCU8CCRsmOrAccelSwt/1  "<pOUTP_bool_HCU8CCRsmOrAccelSwt>"
  Bus_PT_HCU13/15 -> pOUTP_bool_HCU13BatTempWarn/1  "<pOUTP_bool_HCU13BatTempWarn>"
  Bus_PT_HCU13/16 -> pOUTP_bool_HCU13RemanACOnTip/1  "<pOUTP_bool_HCU13RemanACOnTip>"
  Bus_PT_HCU13/17 -> pOUTP_st_HCU13NoiseVoiceCnfig/1  "<pOUTP_st_HCU13NoiseVoiceCnfig>"
  Bus_PT_HCU15/2 -> pOUTP_Nm_HCU15MAMTrq/1  "<pOUTP_Nm_HCU15MAMTrq>"
  Bus_PT_HCU15/1 -> pOUTP_Nm_HCU15ActTrq/1  "<pOUTP_Nm_HCU15ActTrq>"
  pCANR_st_ACC1ACCStACCDecelReq/1 -> Bus Creator9/6  "pCANR_st_ACC1ACCStACCDecelReq"
  pCANR_Nm_ACC1ACCTrqReq/1 -> Bus Creator9/5  "pCANR_Nm_ACC1ACCTrqReq"
  pCANR_st_ACC1ACCStTrqReq/1 -> Bus Creator9/4  "pCANR_st_ACC1ACCStTrqReq"
  pCANR_mps2_ACC1ACCDecelReq/1 -> Bus Creator9/3  "pCANR_mps2_ACC1ACCDecelReq"
  pCANR_st_ACC1ACCSt/1 -> Bus Creator9/2  "pCANR_st_ACC1ACCSt"
  pCANR_st_ACC1ACCErrSt/1 -> Bus Creator9/1  "pCANR_st_ACC1ACCErrSt"
  pCANR_bool_ABS3HHCAvail/1 -> Bus Creator33/8  "pCANR_bool_ABS3HHCAvail"
  Bus Creator36/1 -> Bus Creator44/4  "pCANR_EPB"
  pCANR_st_EPB1EPBSt/1 -> Bus Creator36/1  "pCANR_st_EPB1EPBSt"
  pCANR_bool_EPB1EPBErrSt/1 -> Bus Creator36/2  "pCANR_bool_EPB1EPBErrSt"
  Bus_PT_HCU4/3 -> pOUTP_st_HCU4BrkSwt/1  "<pOUTP_st_HCU4BrkSwt>"
  Bus_PT_HCU4/5 -> pOUTP_bool_HCU4KickDwnReq/1  "<pOUTP_bool_HCU4KickDwnReq>"
  Bus_PT_HCU4/6 -> pOUTP_bool_HCU4ACOnFeedBack/1  "<pOUTP_bool_HCU4ACOnFeedBack>"
  Bus_PT_HCU4/7 -> pOUTP_bool_HCU4AccelPedOvrid/1  "<pOUTP_bool_HCU4AccelPedOvrid>"
  Bus_PT_HCU13/7 -> pOUTP_bool_HCU13TMErrSt/1  "<pOUTP_bool_HCU13TMErrSt>"
  s_TBoxBswErr_na/1 -> Bus Creator/50  "s_TBoxBswErr_na"
  s_ChrgSnsrBswErr_na/1 -> Bus Creator/51  "s_ChrgSnsrBswErr_na"
  s_MotBatEmgcySignalErr_na/1 -> Bus Creator/52  "s_MotBatEmgcySignalErr_na"
  s_EEMBswErr_na/1 -> Bus Creator/53  "s_EEMBswErr_na"
  s_NoiseSimuBswErr_na/1 -> Bus Creator/54  "s_NoiseSimuBswErr_na"
  s_PasvStaCheckBswErr_na/1 -> Bus Creator/55  "s_PasvStaCheckBswErr_na"
  s_PEPSBswErr_na/1 -> Bus Creator/56  "s_PEPSBswErr_na"
  pHWIN_degC_SlowChrgSensr1Temp/1 -> Bus Creator45/18  "pHWIN_degC_SlowChrgSensr1Temp"
  pHWIN_degC_FastChrgSensr1Temp/1 -> Bus Creator45/19  "pHWIN_degC_FastChrgSensr1Temp"
  pHWIN_degC_SlowChrgSensr2Temp/1 -> Bus Creator45/20  "pHWIN_degC_SlowChrgSensr2Temp"
  pHWIN_degC_FastChrgSensr2Temp/1 -> Bus Creator45/21  "pHWIN_degC_FastChrgSensr2Temp"
  pCANR_rpm_MCU11TMSpd/1 -> Bus Creator2/1  "pCANR_rpm_MCU11TMSpd"
  pCANR_Nm_MCU11TMTrq/1 -> Bus Creator2/2  "pCANR_Nm_MCU11TMTrq"
  pCANR_V_MCU11TMCapVolt/1 -> Bus Creator2/3  "pCANR_V_MCU11TMCapVolt"
  pCANR_bool_MCU11TMTrqValid/1 -> Bus Creator2/4  "pCANR_bool_MCU11TMTrqValid"
  pCANR_bool_MCU11PreChrgAllow/1 -> Bus Creator2/5  "pCANR_bool_MCU11PreChrgAllow"
  pCANR_st_MCU11TMSt/1 -> Bus Creator2/6  "pCANR_st_MCU11TMSt"
  pCANR_st_MCU11TMErrSt/1 -> Bus Creator2/7  "pCANR_st_MCU11TMErrSt"
  pCANR_rpm_MCU21TMSpd/1 -> Bus Creator2/9  "pCANR_rpm_MCU21TMSpd"
  pCANR_Nm_MCU21TMTrq/1 -> Bus Creator2/10  "pCANR_Nm_MCU21TMTrq"
  pCANR_V_MCU21TMCapVolt/1 -> Bus Creator2/11  "pCANR_V_MCU21TMCapVolt"
  pCANR_bool_MCU21TMTrqValid/1 -> Bus Creator2/12  "pCANR_bool_MCU21TMTrqValid"
  pCANR_bool_MCU21PreChrgAllow/1 -> Bus Creator2/13  "pCANR_bool_MCU21PreChrgAllow"
  pCANR_st_MCU21TMSt/1 -> Bus Creator2/14  "pCANR_st_MCU21TMSt"
  pCANR_st_MCU21TMErrSt/1 -> Bus Creator2/15  "pCANR_st_MCU21TMErrSt"
  pCANR_Nm_MCU22CalTMTrq/1 -> Bus Creator3/6  "pCANR_Nm_MCU22CalTMTrq"
  pCANR_Nm_MCU22TMMAGTrq/1 -> Bus Creator3/5  "pCANR_Nm_MCU22TMMAGTrq"
  pCANR_Nm_MCU22TMMAMTrq/1 -> Bus Creator3/4  "pCANR_Nm_MCU22TMMAMTrq"
  pCANR_Nm_MCU12CalTMTrq/1 -> Bus Creator3/3  "pCANR_Nm_MCU12CalTMTrq"
  pCANR_Nm_MCU12TMMAMTrq/1 -> Bus Creator3/1  "pCANR_Nm_MCU12TMMAMTrq"
  pCANR_Nm_MCU12TMMAGTrq/1 -> Bus Creator3/2  "pCANR_Nm_MCU12TMMAGTrq"
  pCANR_st_MCU23CoolReq/1 -> Bus Creator13/2  "pCANR_st_MCU23CoolReq"
  pCANR_st_MCU13CoolReq/1 -> Bus Creator13/1  "pCANR_st_MCU13CoolReq"
  Bus Creator2/1 -> Bus Creator4/1  "pCANR_MCU1"
  Bus Creator3/1 -> Bus Creator4/2  "pCANR_MCU2"
  Bus Creator13/1 -> Bus Creator4/3  "pCANR_MCU3"
  Constant29/1 -> Bus Creator/30  "s_AsrIntvVld_na"
  Constant28/1 -> Bus Creator/29  "s_AbsIntvVld_na"
  Constant27/1 -> Bus Creator/28  "s_BrkPedlPVld_na"
  Constant30/1 -> Bus Creator/31  "s_RegenTrqVld_na"
  Constant31/1 -> Bus Creator/32  "s_MsrIntvVld_na"
  pCANR_mps2_YRS2AX1Ofst/1 -> Bus Creator34/1  "pCANR_mps2_YRS2AX1Ofst"
  pCANR_mps2_YRS2AY1Ofst/1 -> Bus Creator34/2  "pCANR_mps2_YRS2AY1Ofst"
  Bus Creator34/1 -> Bus Creator48/2  "pCANR_YRS2"
  pCANR_bool_BCM13DrvDoorSt/1 -> Bus Creator24/1  "pCANR_bool_BCM13DrvDoorSt"
  pCANR_bool_BCM13HighBeamCmd/1 -> Bus Creator24/2  "pCANR_bool_BCM13HighBeamCmd"
  pCANR_st_BCM13WiperStatus/1 -> Bus Creator24/3  "pCANR_st_BCM13WiperStatus"
  Bus Creator24/1 -> Bus Creator44/6  "pCANR_BCM13"
  pCANR_st_EGSM1ErrSt/1 -> Bus Creator26/5  "pCANR_st_EGSM1ErrSt"
  pCANR_st_EGSM1SecBtnSt/1 -> Bus Creator26/4  "pCANR_st_EGSM1SecBtnSt"
  pHWIN_st_EPark/1 -> Bus Creator45/22  "pHWIN_st_EPark"
  pCANR_bool_EparkErrSt/1 -> Bus Creator23/4  "pCANR_bool_EparkErrSt"
  pCANR_Nm_ASR1TrqRdctFastASR1/1 -> Bus Creator27/1  "pCANR_Nm_ASR1TrqRdctFastASR1"
  pCANR_Nm_ASR1TrqIncrsMSR1/1 -> Bus Creator27/2  "pCANR_Nm_ASR1TrqIncrsMSR1"
  pCANR_bool_ASR1StTRFastASR1/1 -> Bus Creator27/3  "pCANR_bool_ASR1StTRFastASR1"
  pCANR_Nm_ASR2TrqRdctFastASR2/1 -> Bus Creator22/1  "pCANR_Nm_ASR2TrqRdctFastASR2"
  pCANR_bool_ASR2StTRFastASR2/1 -> Bus Creator22/3  "pCANR_bool_ASR2StTRFastASR2"
  pCANR_bool_ASR1StTIMSR1/1 -> Bus Creator27/4  "pCANR_bool_ASR1StTIMSR1"
  pCANR_bool_ABS6StRegenTrqReq/1 -> Bus Creator32/2  "pCANR_bool_ABS6StRegenTrqReq"
  pCANR_Nm_ABS6RegenTrqReq/1 -> Bus Creator32/1  "pCANR_Nm_ABS6RegenTrqReq"
  pCANR_Nm_ASR2TrqIncrsMSR2/1 -> Bus Creator22/2  "pCANR_Nm_ASR2TrqIncrsMSR2"
  pCANR_bool_ASR2StTIMSR2/1 -> Bus Creator22/4  "pCANR_bool_ASR2StTIMSR2"
  Bus Creator22/1 -> Bus Creator44/11  "pCANR_ASR2"
  Bus Creator32/1 -> Bus Creator44/12  "pCANR_ABS6"
  Bus Creator48/1 -> Bus Creator44/13  "pCANR_YRS"
  Bus Creator35/1 -> Bus Creator44/14  "pCANR_NoiseSimu1"
  Bus Creator40/1 -> Bus Creator44/15  "pCANR_AC"
  Bus Creator43/1 -> Bus Creator44/16  "pCANR_TBOX"
  Bus Creator9/1 -> Bus Creator44/17  "pCANR_ACC1"
  Bus_PT_HCU18/1 -> pOUTP_Nm_HCU18MCU1ActTMTrq/1  "<pOUTP_Nm_HCU18MCU1ActTMTrq>"
  Bus_PT_HCU18/2 -> pOUTP_Nm_HCU18MCU1MAMTrq/1  "<pOUTP_Nm_HCU18MCU1MAMTrq>"
  Bus_PT_HCU18/3 -> pOUTP_Nm_HCU18MCU1MAGTrq/1  "<pOUTP_Nm_HCU18MCU1MAGTrq>"
  Bus_PT_HCU19/1 -> pOUTP_Nm_HCU19MCU2ActTMTrq/1  "<pOUTP_Nm_HCU19MCU2ActTMTrq>"
  Bus_PT_HCU19/2 -> pOUTP_Nm_HCU19MCU2MAMTrq/1  "<pOUTP_Nm_HCU19MCU2MAMTrq>"
  Bus_PT_HCU19/3 -> pOUTP_Nm_HCU19MCU2MAGTrq/1  "<pOUTP_Nm_HCU19MCU2MAGTrq>"
  pCANR_bool_MCU21ShtdwnAllow/1 -> Bus Creator2/16  "pCANR_bool_MCU21ShtdwnAllow"
  pCANR_bool_MCU11ShtdwnAllow/1 -> Bus Creator2/8  "pCANR_bool_MCU11ShtdwnAllow"
  Bus_PT_HCU18/4 -> pOUTP_rpm_HCU18MCU1MotCtrlActRev/1  "<pOUTP_rpm_HCU18MCU1ActRev>"
  Bus_PT_HCU19/4 -> pOUTP_rpm_HCU19MCU2MotCtrlActRev/1  "<pOUTP_rpm_HCU19MCU2ActRev>"
  pCANR_pct_ABS2BrakePedalPos/1 -> Bus Creator31/4  "pCANR_pct_ABS2BrakePedalPos"
  pCANR_st_ACU1DrvSideBuckSts/1 -> Bus Creator15/3  "pCANR_st_ACU1DrvSideBuckSts"
  Bus_PT_HCU5/6 -> pOUTP_ratio_HCU5AltitudeFac/1  "<pOUTP_ratio_HCU5AltitudeFac>"
  pHWIN_mV_VacAmbientPres/1 -> Bus Creator45/23  "pHWIN_mV_VacAmbientPres"
  Bus_PT_HCU5/1 -> pOUTP_Nm_HCU5IndicateTrqFront/1  "<pOUTP_Nm_HCU5IndicateTrqFront>"
  Bus_PT_HCU5/2 -> pOUTP_Nm_HCU5IndicateTrqRear/1  "<pOUTP_Nm_HCU5IndicateTrqRear>"

== system HQEV_MiL_20160830_integrate/MiL/Test_Integration/IC/IC/Subsystem ==
  In1 : Inport
  Constant : Constant  Value=0
  Constant1 : Constant  Value=0
  Terminator : Terminator
  HandBrakeSt : Outport
  DDSPS : Outport  Port=2
  wires:
  Constant/1 -> HandBrakeSt/1
  Constant1/1 -> DDSPS/1
  In1/1 -> Terminator/1
